simulink model "controlador_hoist"  (R2023b)
settings: Solver=VariableStepAuto  StartTime=0.0  StopTime=10.0  RelTol=1e-3
undefined symbols (not defined in the file): g, ih, J_hd_hEb, J_hm_hb, N_h, omega_h, rhd, Ts2, zitta_h
libraries: simulink x1
settings Model: Creator=Nahuel  LastModifiedBy=nahue

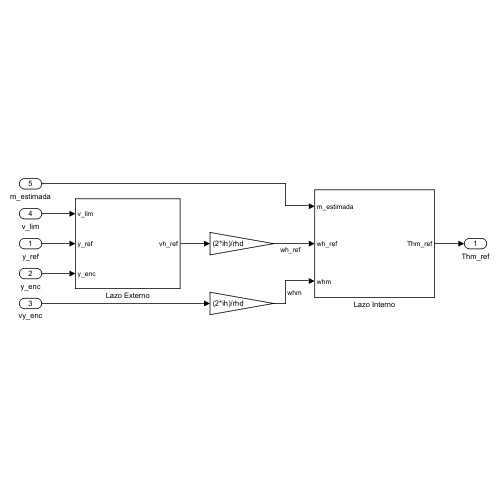
[thumbnail: Simulink's stored preview of the top-level diagram]
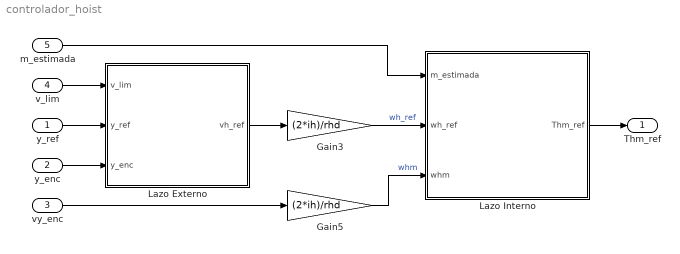
== system controlador_hoist ==
  y_ref : Inport
  y_enc : Inport  Port=2
  vy_enc : Inport  Port=3
  v_lim : Inport  Port=4
  m_estimada : Inport  Port=5
  Gain3 : Gain  Gain=(2*ih)/rhd
  Gain5 : Gain  Gain=(2*ih)/rhd
  Lazo Externo : Subsystem  SystemSampleTime=Ts2
  Lazo Interno : Subsystem  SystemSampleTime=Ts2
  Thm_ref : Outport
  wires:
  vy_enc/1 -> Gain5/1
  Gain3/1 -> Lazo Interno/2(wh_ref)  "wh_ref"
  Gain5/1 -> Lazo Interno/3(whm)  "whm"
  Lazo Interno/1(Thm_ref) -> Thm_ref/1
  y_ref/1 -> Lazo Externo/2(y_ref)
  y_enc/1 -> Lazo Externo/3(y_enc)
  Lazo Externo/1(vh_ref) -> Gain3/1
  v_lim/1 -> Lazo Externo/1(v_lim)
  m_estimada/1 -> Lazo Interno/1(m_estimada)

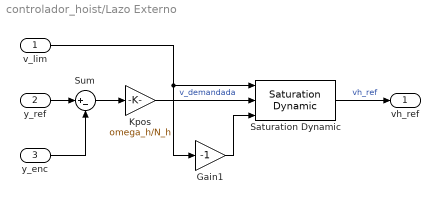
== system controlador_hoist/Lazo Externo ==
  v_lim : Inport
  y_ref : Inport  Port=2
  y_enc : Inport  Port=3
  Gain1 : Gain  Gain=-1
  Kpos : Gain  Gain=omega_h/N_h
  Saturation Dynamic : simulink/Discontinuities/Saturation Dynamic  OutMin=[]  OutMax=[]  OutDataTypeStr=Inherit: Same as second input  OutDataType=fixdt(1, 16)  OutScaling=2^-10  DoSatur=off
  Sum : Sum  Inputs=|+-
  vh_ref : Outport
  wires:
  y_ref/1 -> Sum/1
  v_lim/1 -> Saturation Dynamic/1, Gain1/1
  Gain1/1 -> Saturation Dynamic/3
  y_enc/1 -> Sum/2
  Kpos/1 -> Saturation Dynamic/2  "v_demandada"
  Sum/1 -> Kpos/1
  Saturation Dynamic/1 -> vh_ref/1  "vh_ref"

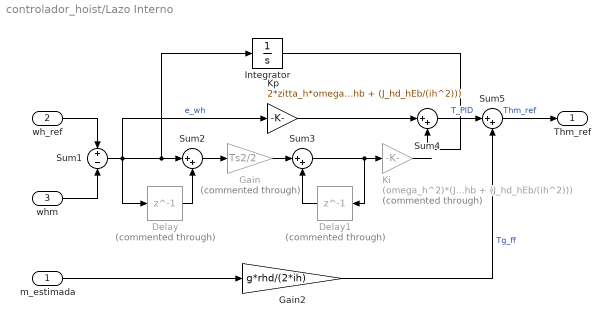
== system controlador_hoist/Lazo Interno ==
  m_estimada : Inport
  wh_ref : Inport  Port=2
  whm : Inport  Port=3
  Delay : Delay  Commented=through  DelayLength=1
  Delay1 : Delay  Commented=through  DelayLength=1
  Gain : Gain  Commented=through  Gain=Ts2/2
  Gain2 : Gain  Gain=g*rhd/(2*ih)
  Integrator : Integrator
  Ki : Gain  Commented=through  Gain=(omega_h^2)*(J_hm_hb + (J_hd_hEb/(ih^2)))
  Kp : Gain  Gain=2*zitta_h*omega_h*(J_hm_hb + (J_hd_hEb/(ih^2)))
  Sum1 : Sum  Inputs=+-
  Sum{2..5} (4 alike) : Sum  Inputs=|++
  Thm_ref : Outport
  wires:
  Gain/1 -> Sum3/1
  Delay1/1 -> Sum3/2
  Kp/1 -> Sum4/1
  Sum1/1 -> Delay/1, Integrator/1, Sum2/1, Kp/1  "e_wh"
  whm/1 -> Sum1/2
  Sum3/1 -> Delay1/1, Ki/1
  Gain2/1 -> Sum5/2  "Tg_ff"
  Delay/1 -> Sum2/2
  Ki/1 -> ?
  Sum5/1 -> Thm_ref/1  "Thm_ref"
  Sum2/1 -> Gain/1
  Sum4/1 -> Sum5/1  "T_PID"
  wh_ref/1 -> Sum1/1
  m_estimada/1 -> Gain2/1
  Integrator/1 -> Sum4/2
